simulink model "ESTS_FRIC_HILO_test"  (R2024b)
settings: Solver=VariableStepAuto  StartTime=0.0  StopTime=10.0  RelTol=1e-3
libraries: ESTS_FRIC_HILO x1
settings Model: Creator=blatak  LastModifiedBy=blatak

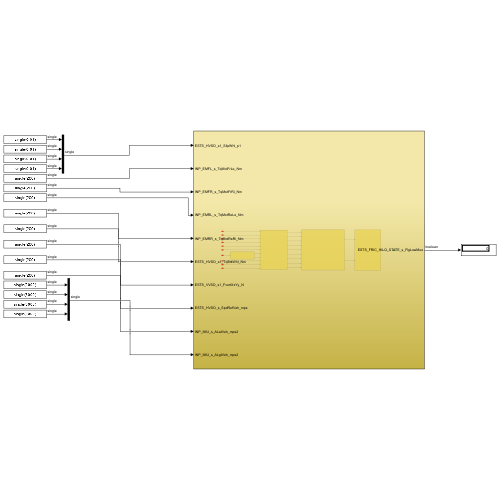
[thumbnail: Simulink's stored preview of the top-level diagram]
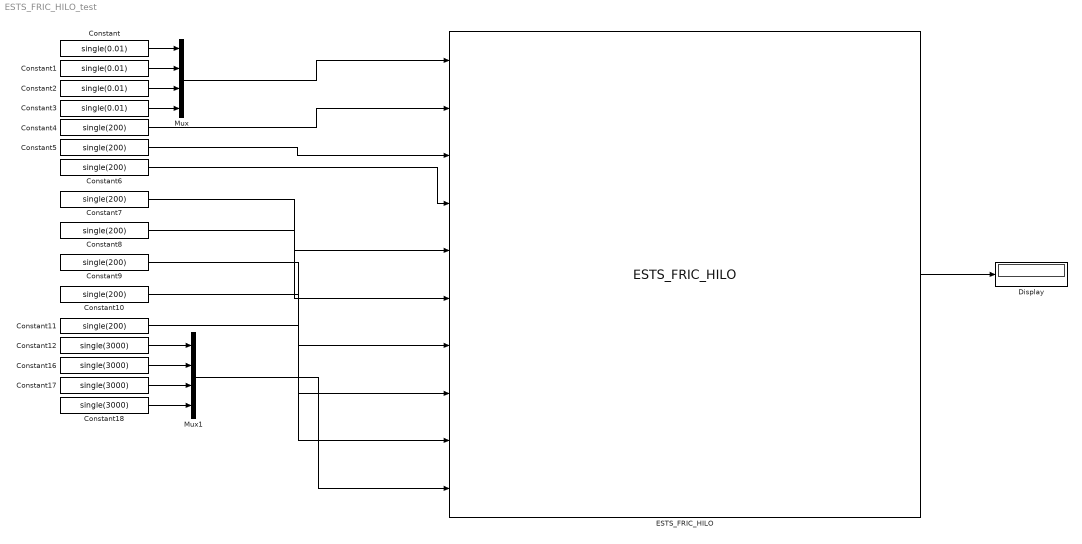
== system ESTS_FRIC_HILO_test ==
  Constant{,1..3} (4 alike) : Constant  Value=single(0.01)
  Constant{4..11} (8 alike) : Constant  Value=single(200)
  Constant{12,16..18} (4 alike) : Constant  Value=single(3000)
  Display : Display
  ESTS_FRIC_HILO : ESTS_FRIC_HILO/ESTS_FRIC_HILO  SystemSampleTime=-1  VariantActivationTime=update diagram  AllowFlexibleInterface=on  Latency=0  AutoFrameSizeCalculation=off
  Mux : Mux
  Mux1 : Mux
  wires:
  Constant8/1 -> ESTS_FRIC_HILO/6
  Constant/1 -> Mux/1
  Constant10/1 -> ESTS_FRIC_HILO/8
  Constant5/1 -> ESTS_FRIC_HILO/3
  Constant9/1 -> ESTS_FRIC_HILO/7
  Constant4/1 -> ESTS_FRIC_HILO/2
  Constant7/1 -> ESTS_FRIC_HILO/5
  Constant3/1 -> Mux/4
  Constant2/1 -> Mux/3
  Constant11/1 -> ESTS_FRIC_HILO/9
  Mux/1 -> ESTS_FRIC_HILO/1
  Constant6/1 -> ESTS_FRIC_HILO/4
  Constant1/1 -> Mux/2
  Constant12/1 -> Mux1/1
  Constant16/1 -> Mux1/2
  Constant17/1 -> Mux1/3
  Constant18/1 -> Mux1/4
  Mux1/1 -> ESTS_FRIC_HILO/10
  ESTS_FRIC_HILO/1 -> Display/1
